simulink model "hdlFrame_Blur_2D_MLFB"  (R2023a)
settings: Solver=VariableStepAuto  StartTime=0.0  StopTime=1  RelTol=1e-3
libraries: visionsources x1
settings Model: Creator=navan  LastModifiedBy=navan
settings SolverCC: MaxZcPerStep=1
settings OptimizationCC: ReuseModelBlockBuffer=off
settings DebuggingCC: UnconnectedInputMsg=warning  UnconnectedOutputMsg=warning  UnconnectedLineMsg=warning  SFMachineParentedDataDiag=error
settings ModelReferenceCC: EnableRefExpFcnMdlSchedulingChecks=on
settings RTWCC: DLArmComputeVersion=19.05

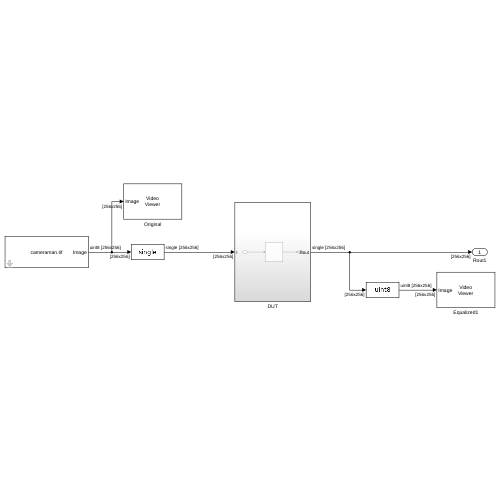
[thumbnail: Simulink's stored preview of the top-level diagram]
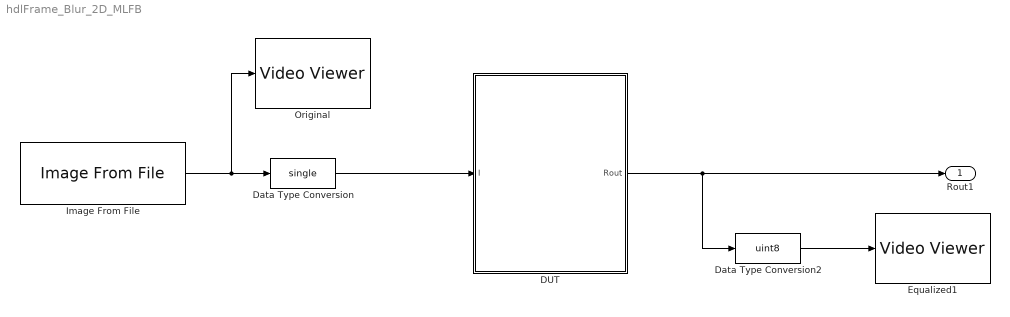
== system hdlFrame_Blur_2D_MLFB ==
  DUT : Subsystem
  Data Type Conversion : DataTypeConversion  OutDataTypeStr=single  SaturateOnIntegerOverflow=off  RndMeth=Floor
  Data Type Conversion2 : DataTypeConversion  OutDataTypeStr=uint8  SaturateOnIntegerOverflow=off  RndMeth=Floor
  Equalized1 : VideoViewer  FigPos=[593 1000 418 304]
  Image From File : visionsources/Image From File  Tag=vipblks_nd  FileName=cameraman.tif  Ts=1  imagePorts=One multidimensional signal  OutPortLabels=R|G|B  ImageDataType=uint8  sdImageDataType=uint(8)  Signed=on  WordLength=16  FractionLengthMode=User-defined  FractionLength=15
  Original : VideoViewer  FigPos=[172 1000 418 304]
  Rout1 : Outport
  wires:
  Data Type Conversion/1 -> DUT/1(I)
  Image From File/1 -> Data Type Conversion/1, Original/1
  Data Type Conversion2/1 -> Equalized1/1
  DUT/1(Rout) -> Rout1/1, Data Type Conversion2/1

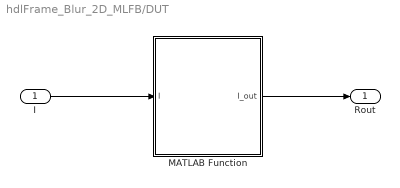
== system hdlFrame_Blur_2D_MLFB/DUT ==
  I : Inport
  MATLAB Function : MATLAB Function  TreatAsAtomicUnit=on
  Rout : Outport
  wires:
  I/1 -> MATLAB Function/1(I)
  MATLAB Function/1(I_out) -> Rout/1

== matlab function hdlFrame_Blur_2D_MLFB/DUT/MATLAB Function ==
  data: I input; I_out output
function I_out = image_blur(I)
% Blur input image

I_out = hdl.npufun(@blur, [3 3], I);

end

function y = blur(N)

y = sum(N(:),'native')/9;

end
